simulink model "ep_5_1"  (R2023b)
settings: Solver=VariableStepAuto  StartTime=0.0  StopTime=10.0  RelTol=1e-3
settings Model: Creator=86186  LastModifiedBy=86186

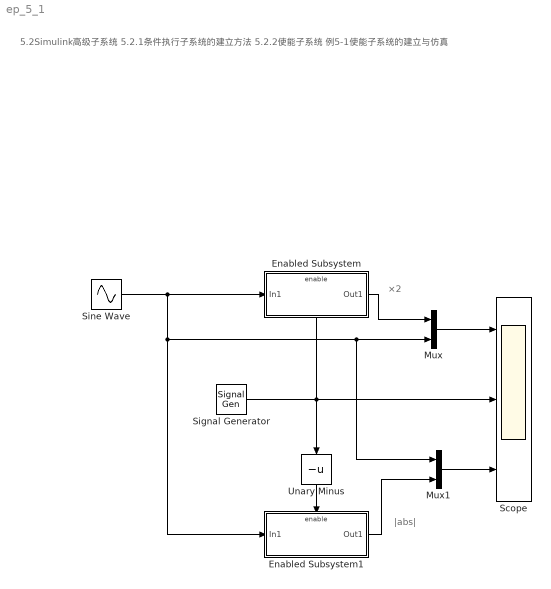
== system ep_5_1 ==
  note: ×2
  note: |abs|
  note: 5.2Simulink高级子系统
      | 5.2.1条件执行子系统的建立方法
      | 5.2.2使能子系统
      | 例5-1使能子系统的建立与仿真
  Enabled Subsystem : Subsystem  TreatAsAtomicUnit=on
  Enabled Subsystem1 : Subsystem  TreatAsAtomicUnit=on
  Mux : Mux  Inputs=2
  Mux1 : Mux  Inputs=2
  Scope : Scope  NumInputPorts=3
  Signal Generator : SignalGenerator  WaveForm=square
  Sine Wave : Sin  SampleTime=0
  Unary Minus : UnaryMinus
  wires:
  Sine Wave/1 -> Enabled Subsystem/1(In1), Mux1/1, Mux/2, Enabled Subsystem1/1(In1)
  Signal Generator/1 -> Enabled Subsystem/Enable, Unary Minus/1, Scope/2
  Unary Minus/1 -> Enabled Subsystem1/Enable
  Enabled Subsystem/1(Out1) -> Mux/1
  Mux/1 -> Scope/1
  Enabled Subsystem1/1(Out1) -> Mux1/2
  Mux1/1 -> Scope/3

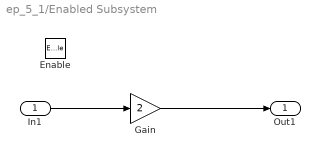
== system ep_5_1/Enabled Subsystem ==
  In1 : Inport
  Enable : EnablePort  StatesWhenEnabling=reset
  Gain : Gain  Gain=2
  Out1 : Outport
  wires:
  In1/1 -> Gain/1
  Gain/1 -> Out1/1

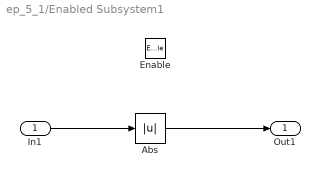
== system ep_5_1/Enabled Subsystem1 ==
  In1 : Inport
  Enable : EnablePort
  Abs : Abs  SaturateOnIntegerOverflow=off
  Out1 : Outport
  wires:
  In1/1 -> Abs/1
  Abs/1 -> Out1/1
